simulink model "ClosedLoop_V1_2020b"  (R2020b)
settings: Solver=ode4  StartTime=0.0  StopTime=TMax  FixedStep=DT  MaxStep=DT  RelTol=1e-3  EnableMultiTasking=on
undefined symbols (not defined in the file or in its folder): CertificationSettings, Control, DiscIntNeverNeededParam, Drivetrain, OutList, P_InitAngle, RPM_Init, sigbuilder_block, SimConfig, strmatch
libraries: simulink x10, simulink_extras x4
(part 2 of 2)

== system ClosedLoop_V1_2020b/Plot aerodynamic Data/Plot Reynolds number ==
  note: B1N1Re      Reynolds number (in millions) at Blade 1, Node 1
      | B1N2Re      Reynolds number (in millions) at Blade 1, Node 2
      | B1N3Re      Reynolds number (in millions) at Blade 1, Node 3
      | B1N4Re      Reynolds number (in millions) at Blade 1, Node 4
      | B1N5Re      Reynolds number (in millions) at Blade 1, Node 5
      | B1N6Re      Reynolds number (in millions) at Blade 1, Node 6
      | B1N7Re      Reynolds number (in millions) at Blade 1, Node 7
      | B1N8Re      Reynolds number (in millions) at Blade 1, Node 8
      | B1N9Re      Reynolds number (in millions) at Blade 1, Node 9
  OutData1 : Inport
  Scope : Scope  NumInputPorts=9
  "extract Reynolds number (in millions) at Blade 1, Node 1" : Fcn  Expr=u(strmatch('B1N1Re',OutList))
  "extract Reynolds number (in millions) at Blade 1, Node 2" : Fcn  Expr=u(strmatch('B1N2Re',OutList))
  "extract Reynolds number (in millions) at Blade 1, Node 3" : Fcn  Expr=u(strmatch('B1N3Re',OutList))
  "extract Reynolds number (in millions) at Blade 1, Node 4" : Fcn  Expr=u(strmatch('B1N4Re',OutList))
  "extract Reynolds number (in millions) at Blade 1, Node 5" : Fcn  Expr=u(strmatch('B1N5Re',OutList))
  "extract Reynolds number (in millions) at Blade 1, Node 6" : Fcn  Expr=u(strmatch('B1N6Re',OutList))
  "extract Reynolds number (in millions) at Blade 1, Node 7" : Fcn  Expr=u(strmatch('B1N7Re',OutList))
  "extract Reynolds number (in millions) at Blade 1, Node 8" : Fcn  Expr=u(strmatch('B1N8Re',OutList))
  "extract Reynolds number (in millions) at Blade 1, Node 9" : Fcn  Expr=u(strmatch('B1N9Re',OutList))
  wires:
  OutData1/1 -> "extract Reynolds number (in millions) at Blade 1, Node 9"/1, "extract Reynolds number (in millions) at Blade 1, Node 8"/1, "extract Reynolds number (in millions) at Blade 1, Node 7"/1, "extract Reynolds number (in millions) at Blade 1, Node 6"/1, "extract Reynolds number (in millions) at Blade 1, Node 5"/1, "extract Reynolds number (in millions) at Blade 1, Node 4"/1, "extract Reynolds number (in millions) at Blade 1, Node 3"/1, "extract Reynolds number (in millions) at Blade 1, Node 2"/1, "extract Reynolds number (in millions) at Blade 1, Node 1"/1
  "extract Reynolds number (in millions) at Blade 1, Node 8"/1 -> Scope/8  "Reynolds number (in millions) at Blade 1, Node 8"
  "extract Reynolds number (in millions) at Blade 1, Node 3"/1 -> Scope/3  "Reynolds number (in millions) at Blade 1, Node 3"
  "extract Reynolds number (in millions) at Blade 1, Node 5"/1 -> Scope/5  "Reynolds number (in millions) at Blade 1, Node 5"
  "extract Reynolds number (in millions) at Blade 1, Node 7"/1 -> Scope/7  "Reynolds number (in millions) at Blade 1, Node 7"
  "extract Reynolds number (in millions) at Blade 1, Node 1"/1 -> Scope/1  "Reynolds number (in millions) at Blade 1, Node 1"
  "extract Reynolds number (in millions) at Blade 1, Node 6"/1 -> Scope/6  "Reynolds number (in millions) at Blade 1, Node 6"
  "extract Reynolds number (in millions) at Blade 1, Node 4"/1 -> Scope/4  "Reynolds number (in millions) at Blade 1, Node 4"
  "extract Reynolds number (in millions) at Blade 1, Node 9"/1 -> Scope/9  "Reynolds number (in millions) at Blade 1, Node 9"
  "extract Reynolds number (in millions) at Blade 1, Node 2"/1 -> Scope/2  "Reynolds number (in millions) at Blade 1, Node 2"

== system ClosedLoop_V1_2020b/Plot aerodynamic Data/Plot Rotor Data ==
  note: RtAeroFxh   Total rotor aerodynamic load (force in x direction) the hub coordinate system N
      | RtAeroFyh   Total rotor aerodynamic load (force in y direction) the hub coordinate system N
      | RtAeroFzh   Total rotor aerodynamic load (force in z direction) the hub coordinate system N
      | RtAeroMxh   Total rotor aerodynamic load (moment in x direction) the hub coordinate system Nm
      | RtAeroMyh   Total rotor aerodynamic load (moment in y direction) the hub coordinate system Nm
      | RtAeroMzh   Total rotor aerodynamic load (moment in z direction) the hub coordinate system Nm
      | RtAeroPwr   Rotor aerodynamic power W
      | RtAeroCp    Rotor aerodynamic power coefficient
      | RtAeroCq    Rotor aerodynamic torque coefficient
      | RtAeroCt    Rotor aerodynamic thrust coefficient
  OutData : Inport
  Scope : Scope  NumInputPorts=3
  Scope1 : Scope  NumInputPorts=3
  Scope{2..5} (4 alike) : Scope
  extract Rotor aerodynamic power W : Fcn  Expr=u(strmatch('RtAeroPwr',OutList))
  extract Rotor aerodynamic power coefficient : Fcn  Expr=u(strmatch('RtAeroCp',OutList))
  extract Rotor aerodynamic thrust coefficient : Fcn  Expr=u(strmatch('RtAeroCt',OutList))
  extract Rotor aerodynamic torque coefficient : Fcn  Expr=u(strmatch('RtAeroCp',OutList))
  extract Total rotor aerodynamic load (force in x direction) hub coordinate system (N) : Fcn  Expr=u(strmatch('RtAeroFxh',OutList))
  extract Total rotor aerodynamic load (force in y direction) hub coordinate system (N) : Fcn  Expr=u(strmatch('RtAeroFyh',OutList))
  extract Total rotor aerodynamic load (force in z direction) hub coordinate system (N) : Fcn  Expr=u(strmatch('RtAeroFzh',OutList))
  extract Total rotor aerodynamic load (moment in x direction) the hub coordinate system Nm : Fcn  Expr=u(strmatch('RtAeroMxh',OutList))
  extract Total rotor aerodynamic load (moment in y direction) the hub coordinate system Nm : Fcn  Expr=u(strmatch('RtAeroMyh',OutList))
  extract Total rotor aerodynamic load (moment in z direction) the hub coordinate system Nm : Fcn  Expr=u(strmatch('RtAeroMzh',OutList))
  wires:
  extract Total rotor aerodynamic load (force in x direction) hub coordinate system (N)/1 -> Scope/1  "Total rotor aerodynamic load (force in x direction) hub coordinate system (N)"
  OutData/1 -> extract Rotor aerodynamic thrust coefficient/1, extract Rotor aerodynamic torque coefficient/1, extract Rotor aerodynamic power coefficient/1, extract Rotor aerodynamic power W/1, extract Total rotor aerodynamic load (moment in z direction) the hub coordinate system Nm/1, extract Total rotor aerodynamic load (moment in y direction) the hub coordinate system Nm/1, extract Total rotor aerodynamic load (force in z direction) hub coordinate system (N)/1, extract Total rotor aerodynamic load (force in y direction) hub coordinate system (N)/1, extract Total rotor aerodynamic load (force in x direction) hub coordinate system (N)/1, extract Total rotor aerodynamic load (moment in x direction) the hub coordinate system Nm/1
  extract Total rotor aerodynamic load (force in y direction) hub coordinate system (N)/1 -> Scope/2  "Total rotor aerodynamic load (force in y direction) hub coordinate system (N)"
  extract Total rotor aerodynamic load (force in z direction) hub coordinate system (N)/1 -> Scope/3  "Total rotor aerodynamic load (force in z direction) hub coordinate system (N)"
  extract Total rotor aerodynamic load (moment in x direction) the hub coordinate system Nm/1 -> Scope1/1  "Total rotor aerodynamic load (moment in x direction) the hub coordinate system Nm"
  extract Total rotor aerodynamic load (moment in y direction) the hub coordinate system Nm/1 -> Scope1/2  "Total rotor aerodynamic load (moment in y direction) the hub coordinate system Nm"
  extract Total rotor aerodynamic load (moment in z direction) the hub coordinate system Nm/1 -> Scope1/3  "Total rotor aerodynamic load (moment in z direction) the hub coordinate system Nm"
  extract Rotor aerodynamic power W/1 -> Scope2/1  "Rotor aerodynamic power W"
  extract Rotor aerodynamic power coefficient/1 -> Scope3/1  "Rotor aerodynamic power coefficient"
  extract Rotor aerodynamic torque coefficient/1 -> Scope4/1  "Rotor aerodynamic torque coefficient"
  extract Rotor aerodynamic thrust coefficient/1 -> Scope5/1  "Rotor aerodynamic thrust coefficient"

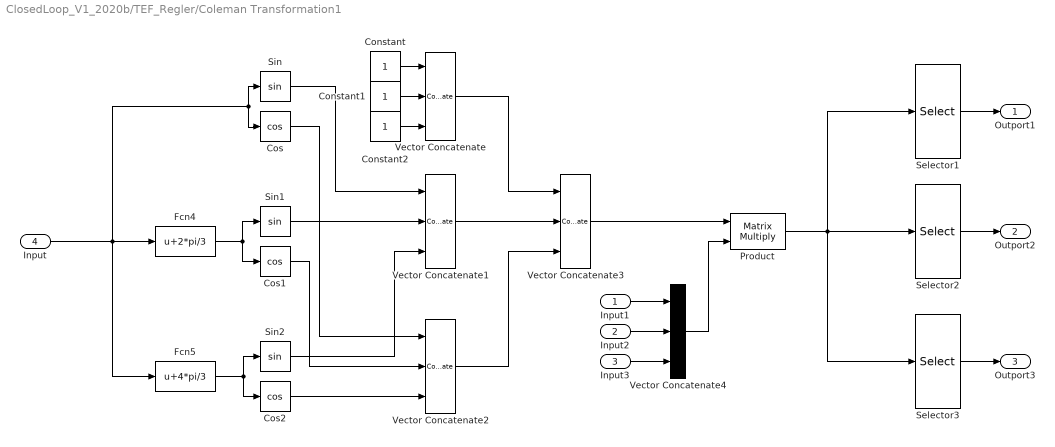
== system ClosedLoop_V1_2020b/TEF_Regler/Coleman Transformation1 ==
  Input1 : Inport
  Input2 : Inport  Port=2
  Input3 : Inport  Port=3
  Input : Inport  Port=4
  Constant : Constant
  Constant1 : Constant
  Constant2 : Constant
  Cos : Trigonometry  Operator=cos
  Cos1 : Trigonometry  Operator=cos
  Cos2 : Trigonometry  Operator=cos
  Fcn4 : Fcn  Expr=u+2*pi/3
  Fcn5 : Fcn  Expr=u+4*pi/3
  Product : Product  Multiplication=Matrix(*)
  Selector1 : Selector  InputPortWidth=3  IndexOptions=Index vector (dialog)  Indices=[1]  OutputSizes=1
  Selector2 : Selector  InputPortWidth=3  IndexOptions=Index vector (dialog)  Indices=[2]  OutputSizes=1
  Selector3 : Selector  InputPortWidth=3  IndexOptions=Index vector (dialog)  Indices=[3]  OutputSizes=1
  Sin : Trigonometry
  Sin1 : Trigonometry
  Sin2 : Trigonometry
  Vector Concatenate{,1..2,4} (4 alike) : Concatenate  NumInputs=3
  Vector Concatenate3 : Concatenate  NumInputs=3  Mode=Multidimensional array  ConcatenateDimension=2
  Outport1 : Outport  VectorParamsAs1DForOutWhenUnconnected=off
  Outport2 : Outport  Port=2  VectorParamsAs1DForOutWhenUnconnected=off
  Outport3 : Outport  Port=3  VectorParamsAs1DForOutWhenUnconnected=off
  wires:
  Input3/1 -> Vector Concatenate4/3
  Input2/1 -> Vector Concatenate4/2
  Input1/1 -> Vector Concatenate4/1
  Constant2/1 -> Vector Concatenate/3
  Vector Concatenate3/1 -> Product/1
  Fcn4/1 -> Cos1/1, Sin1/1
  Vector Concatenate2/1 -> Vector Concatenate3/3
  Selector3/1 -> Outport3/1
  Selector2/1 -> Outport2/1
  Selector1/1 -> Outport1/1
  Vector Concatenate4/1 -> Product/2
  Vector Concatenate1/1 -> Vector Concatenate3/2
  Input/1 -> Cos/1, Sin/1, Fcn4/1, Fcn5/1
  Constant/1 -> Vector Concatenate/1
  Constant1/1 -> Vector Concatenate/2
  Sin2/1 -> Vector Concatenate1/3
  Cos1/1 -> Vector Concatenate2/2
  Cos/1 -> Vector Concatenate2/1
  Sin1/1 -> Vector Concatenate1/2
  Cos2/1 -> Vector Concatenate2/3
  Sin/1 -> Vector Concatenate1/1
  Product/1 -> Selector1/1, Selector2/1, Selector3/1
  Vector Concatenate/1 -> Vector Concatenate3/1
  Fcn5/1 -> Cos2/1, Sin2/1

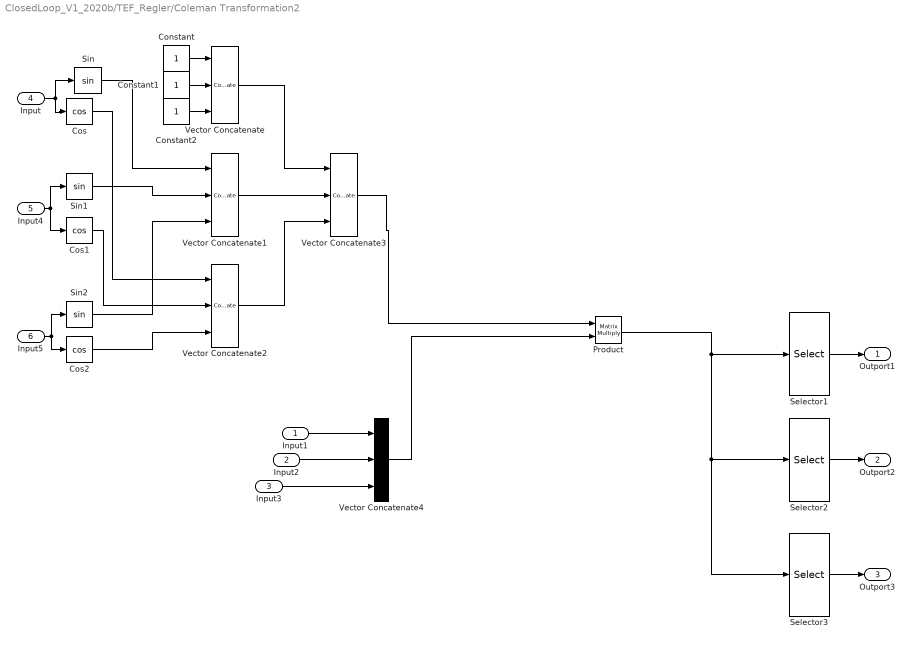
== system ClosedLoop_V1_2020b/TEF_Regler/Coleman Transformation2 ==
  Input1 : Inport
  Input2 : Inport  Port=2
  Input3 : Inport  Port=3
  Input : Inport  Port=4
  Input4 : Inport  Port=5
  Input5 : Inport  Port=6
  Constant : Constant
  Constant1 : Constant
  Constant2 : Constant
  Cos : Trigonometry  Operator=cos
  Cos1 : Trigonometry  Operator=cos
  Cos2 : Trigonometry  Operator=cos
  Product : Product  Multiplication=Matrix(*)
  Selector1 : Selector  InputPortWidth=3  IndexOptions=Index vector (dialog)  Indices=[1]  OutputSizes=1
  Selector2 : Selector  InputPortWidth=3  IndexOptions=Index vector (dialog)  Indices=[2]  OutputSizes=1
  Selector3 : Selector  InputPortWidth=3  IndexOptions=Index vector (dialog)  Indices=[3]  OutputSizes=1
  Sin : Trigonometry
  Sin1 : Trigonometry
  Sin2 : Trigonometry
  Vector Concatenate{,1..2,4} (4 alike) : Concatenate  NumInputs=3
  Vector Concatenate3 : Concatenate  NumInputs=3  Mode=Multidimensional array  ConcatenateDimension=2
  Outport1 : Outport  VectorParamsAs1DForOutWhenUnconnected=off
  Outport2 : Outport  Port=2  VectorParamsAs1DForOutWhenUnconnected=off
  Outport3 : Outport  Port=3  VectorParamsAs1DForOutWhenUnconnected=off
  wires:
  Input3/1 -> Vector Concatenate4/3
  Input2/1 -> Vector Concatenate4/2
  Input1/1 -> Vector Concatenate4/1
  Constant2/1 -> Vector Concatenate/3
  Vector Concatenate3/1 -> Product/1
  Input4/1 -> Sin1/1, Cos1/1
  Vector Concatenate2/1 -> Vector Concatenate3/3
  Selector3/1 -> Outport3/1
  Selector2/1 -> Outport2/1
  Selector1/1 -> Outport1/1
  Vector Concatenate4/1 -> Product/2
  Vector Concatenate1/1 -> Vector Concatenate3/2
  Input5/1 -> Sin2/1, Cos2/1
  Constant/1 -> Vector Concatenate/1
  Constant1/1 -> Vector Concatenate/2
  Sin2/1 -> Vector Concatenate1/3
  Cos1/1 -> Vector Concatenate2/2
  Cos/1 -> Vector Concatenate2/1
  Sin1/1 -> Vector Concatenate1/2
  Cos2/1 -> Vector Concatenate2/3
  Sin/1 -> Vector Concatenate1/1
  Input/1 -> Sin/1, Cos/1
  Product/1 -> Selector1/1, Selector2/1, Selector3/1
  Vector Concatenate/1 -> Vector Concatenate3/1

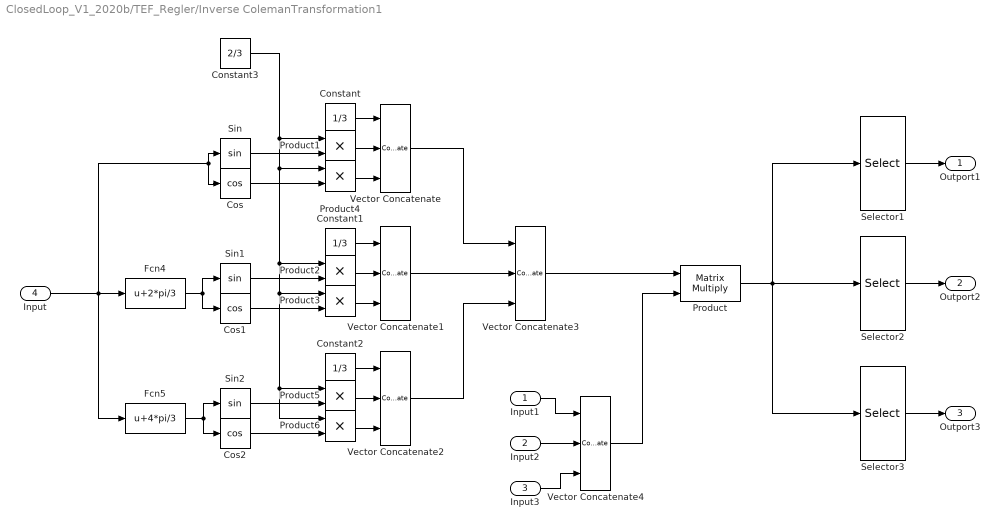
== system ClosedLoop_V1_2020b/TEF_Regler/Inverse ColemanTransformation1 ==
  Input1 : Inport
  Input2 : Inport  Port=2
  Input3 : Inport  Port=3
  Input : Inport  Port=4
  Constant : Constant  Value=1/3
  Constant1 : Constant  Value=1/3
  Constant2 : Constant  Value=1/3
  Constant3 : Constant  Value=2/3
  Cos : Trigonometry  Operator=cos
  Cos1 : Trigonometry  Operator=cos
  Cos2 : Trigonometry  Operator=cos
  Fcn4 : Fcn  Expr=u+2*pi/3
  Fcn5 : Fcn  Expr=u+4*pi/3
  Product : Product  Multiplication=Matrix(*)
  Product{1..6} (6 alike) : Product
  Selector1 : Selector  InputPortWidth=3  IndexOptions=Index vector (dialog)  Indices=[1]  OutputSizes=1
  Selector2 : Selector  InputPortWidth=3  IndexOptions=Index vector (dialog)  Indices=[2]  OutputSizes=1
  Selector3 : Selector  InputPortWidth=3  IndexOptions=Index vector (dialog)  Indices=[3]  OutputSizes=1
  Sin : Trigonometry
  Sin1 : Trigonometry
  Sin2 : Trigonometry
  Vector Concatenate{,1..2,4} (4 alike) : Concatenate  NumInputs=3  Mode=Multidimensional array
  Vector Concatenate3 : Concatenate  NumInputs=3  Mode=Multidimensional array  ConcatenateDimension=2
  Outport1 : Outport  VectorParamsAs1DForOutWhenUnconnected=off
  Outport2 : Outport  Port=2  VectorParamsAs1DForOutWhenUnconnected=off
  Outport3 : Outport  Port=3  VectorParamsAs1DForOutWhenUnconnected=off
  wires:
  Selector2/1 -> Outport2/1
  Selector3/1 -> Outport3/1
  Product/1 -> Selector1/1, Selector2/1, Selector3/1
  Selector1/1 -> Outport1/1
  Product2/1 -> Vector Concatenate1/2
  Product1/1 -> Vector Concatenate/2
  Constant/1 -> Vector Concatenate/1
  Vector Concatenate1/1 -> Vector Concatenate3/2
  Vector Concatenate2/1 -> Vector Concatenate3/3
  Vector Concatenate/1 -> Vector Concatenate3/1
  Vector Concatenate3/1 -> Product/1
  Input/1 -> Fcn4/1, Fcn5/1, Cos/1, Sin/1
  Product4/1 -> Vector Concatenate/3
  Sin1/1 -> Product2/2
  Constant1/1 -> Vector Concatenate1/1
  Product6/1 -> Vector Concatenate2/3
  Constant2/1 -> Vector Concatenate2/1
  Product3/1 -> Vector Concatenate1/3
  Sin/1 -> Product1/2
  Product5/1 -> Vector Concatenate2/2
  Input3/1 -> Vector Concatenate4/3
  Vector Concatenate4/1 -> Product/2
  Input1/1 -> Vector Concatenate4/1
  Input2/1 -> Vector Concatenate4/2
  Constant3/1 -> Product4/1, Product2/1, Product6/1, Product5/1, Product3/1, Product1/1
  Cos/1 -> Product4/2
  Cos1/1 -> Product3/2
  Sin2/1 -> Product5/2
  Cos2/1 -> Product6/2
  Fcn4/1 -> Sin1/1, Cos1/1
  Fcn5/1 -> Sin2/1, Cos2/1

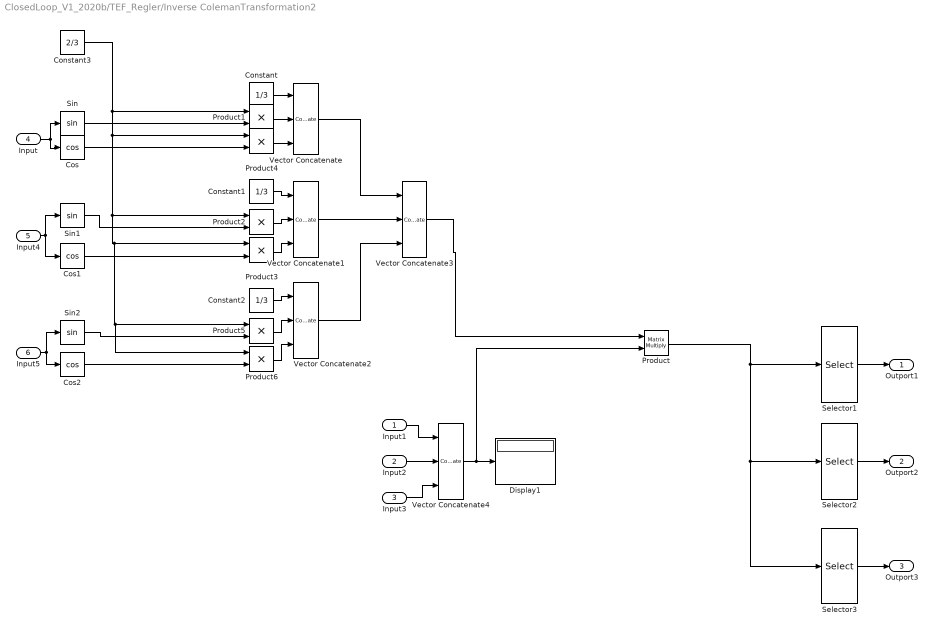
== system ClosedLoop_V1_2020b/TEF_Regler/Inverse ColemanTransformation2 ==
  Input1 : Inport
  Input2 : Inport  Port=2
  Input3 : Inport  Port=3
  Input : Inport  Port=4
  Input4 : Inport  Port=5
  Input5 : Inport  Port=6
  Constant : Constant  Value=1/3
  Constant1 : Constant  Value=1/3
  Constant2 : Constant  Value=1/3
  Constant3 : Constant  Value=2/3
  Cos : Trigonometry  Operator=cos
  Cos1 : Trigonometry  Operator=cos
  Cos2 : Trigonometry  Operator=cos
  Display1 : Display
  Product : Product  Multiplication=Matrix(*)
  Product{1..6} (6 alike) : Product
  Selector1 : Selector  InputPortWidth=3  IndexOptions=Index vector (dialog)  Indices=[1]  OutputSizes=1
  Selector2 : Selector  InputPortWidth=3  IndexOptions=Index vector (dialog)  Indices=[2]  OutputSizes=1
  Selector3 : Selector  InputPortWidth=3  IndexOptions=Index vector (dialog)  Indices=[3]  OutputSizes=1
  Sin : Trigonometry
  Sin1 : Trigonometry
  Sin2 : Trigonometry
  Vector Concatenate{,1..2,4} (4 alike) : Concatenate  NumInputs=3  Mode=Multidimensional array
  Vector Concatenate3 : Concatenate  NumInputs=3  Mode=Multidimensional array  ConcatenateDimension=2
  Outport1 : Outport  VectorParamsAs1DForOutWhenUnconnected=off
  Outport2 : Outport  Port=2  VectorParamsAs1DForOutWhenUnconnected=off
  Outport3 : Outport  Port=3  VectorParamsAs1DForOutWhenUnconnected=off
  wires:
  Selector2/1 -> Outport2/1
  Selector3/1 -> Outport3/1
  Product/1 -> Selector1/1, Selector2/1, Selector3/1
  Selector1/1 -> Outport1/1
  Input4/1 -> Sin1/1, Cos1/1
  Product2/1 -> Vector Concatenate1/2
  Product1/1 -> Vector Concatenate/2
  Constant/1 -> Vector Concatenate/1
  Vector Concatenate1/1 -> Vector Concatenate3/2
  Vector Concatenate2/1 -> Vector Concatenate3/3
  Input/1 -> Cos/1, Sin/1
  Vector Concatenate/1 -> Vector Concatenate3/1
  Vector Concatenate3/1 -> Product/1
  Input5/1 -> Sin2/1, Cos2/1
  Product4/1 -> Vector Concatenate/3
  Sin1/1 -> Product2/2
  Constant1/1 -> Vector Concatenate1/1
  Product6/1 -> Vector Concatenate2/3
  Constant2/1 -> Vector Concatenate2/1
  Product3/1 -> Vector Concatenate1/3
  Sin/1 -> Product1/2
  Product5/1 -> Vector Concatenate2/2
  Input3/1 -> Vector Concatenate4/3
  Vector Concatenate4/1 -> Display1/1, Product/2
  Input1/1 -> Vector Concatenate4/1
  Input2/1 -> Vector Concatenate4/2
  Constant3/1 -> Product1/1, Product4/1, Product2/1, Product3/1, Product5/1, Product6/1
  Cos/1 -> Product4/2
  Cos1/1 -> Product3/2
  Sin2/1 -> Product5/2
  Cos2/1 -> Product6/2

== system ClosedLoop_V1_2020b/TEF_Regler/Subsystem ==
  In1 : Inport
  Derivative : Derivative
  Gain : Gain  Gain=SimConfig.controller.TEF.K_P
  Gain1 : Gain  Gain=SimConfig.controller.TEF.K_I
  Gain2 : Gain  Gain=SimConfig.controller.TEF.K_D
  Integrator : Integrator
  Scope : Scope  NumInputPorts=2
  Scope1 : Scope  NumInputPorts=2
  Scope2 : Scope  NumInputPorts=5
  Sum : Sum  Inputs=+++
  Out1 : Outport  VectorParamsAs1DForOutWhenUnconnected=off
  wires:
  Sum/1 -> Scope2/4, Out1/1
  Integrator/1 -> Gain1/1  "I"
  Derivative/1 -> Gain2/1
  In1/1 -> Scope2/5, Scope/1, Gain/1, Scope1/2, Integrator/1, Derivative/1
  Gain/1 -> Scope/2, Scope2/2, Sum/2  "P"
  Gain1/1 -> Scope1/1, Scope2/3, Sum/3
  Gain2/1 -> Sum/1, Scope2/1  "D"

== system ClosedLoop_V1_2020b/TEF_Regler/Subsystem1 ==
  In1 : Inport
  Derivative : Derivative
  Gain : Gain  Gain=SimConfig.controller.TEF.K_P
  Gain1 : Gain  Gain=SimConfig.controller.TEF.K_I
  Gain2 : Gain  Gain=SimConfig.controller.TEF.K_D
  Integrator : Integrator
  Sum : Sum  Inputs=+++
  Out1 : Outport  VectorParamsAs1DForOutWhenUnconnected=off
  wires:
  Gain2/1 -> Sum/1
  Gain1/1 -> Sum/3
  Gain/1 -> Sum/2
  In1/1 -> Derivative/1, Integrator/1, Gain/1
  Derivative/1 -> Gain2/1
  Integrator/1 -> Gain1/1
  Sum/1 -> Out1/1

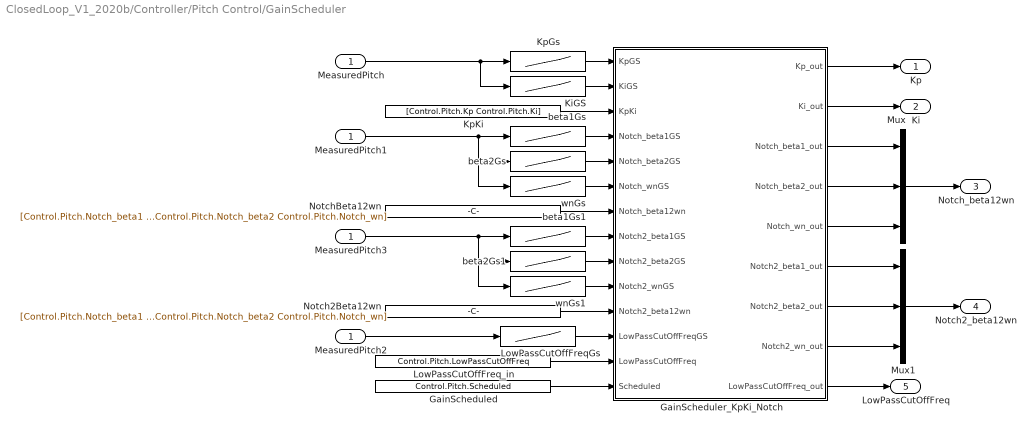
== system ClosedLoop_V1_2020b/Controller/Pitch Control/GainScheduler ==
  MeasuredPitch : Inport
  GainScheduled : Constant  Value=Control.Pitch.Scheduled
  GainScheduler_KpKi_Notch : MATLAB Function  TreatAsAtomicUnit=on
  KiGS : Lookup_n-D  NumberOfTableDimensions=1  BreakpointsForDimension1=Control.Pitch.ScheduledPitchAngles  Table=Control.Pitch.KiGS  ExtrapMethod=Clip  UseLastTableValue=on  InternalRulePriority=Speed  RndMeth=Simplest  InputSameDT=on
  KpGs : Lookup_n-D  NumberOfTableDimensions=1  BreakpointsForDimension1=Control.Pitch.ScheduledPitchAngles  Table=Control.Pitch.KpGS  ExtrapMethod=Clip  UseLastTableValue=on  InternalRulePriority=Speed  RndMeth=Simplest  InputSameDT=on
  KpKi : Constant  Value=[Control.Pitch.Kp Control.Pitch.Ki]
  LowPassCutOffFreqGs : Lookup_n-D  NumberOfTableDimensions=1  BreakpointsForDimension1=Control.Pitch.ScheduledPitchAngles  Table=Control.Pitch.LowPassCutOffFreqGS  ExtrapMethod=Clip  UseLastTableValue=on  InternalRulePriority=Speed  RndMeth=Simplest  InputSameDT=on
  LowPassCutOffFreq_in : Constant  Value=Control.Pitch.LowPassCutOffFreq
  MeasuredPitch1 : InportShadow
  MeasuredPitch2 : InportShadow
  MeasuredPitch3 : InportShadow
  Mux : Mux  Inputs=3
  Mux1 : Mux  Inputs=3
  Notch2Beta12wn : Constant  Value=[Control.Pitch.Notch_beta1 Control.Pitch.Notch_beta2 Control.Pitch.Notch_wn]
  NotchBeta12wn : Constant  Value=[Control.Pitch.Notch_beta1 Control.Pitch.Notch_beta2 Control.Pitch.Notch_wn]
  beta1Gs : Lookup_n-D  NumberOfTableDimensions=1  BreakpointsForDimension1=Control.Pitch.ScheduledPitchAngles  Table=Control.Pitch.Notch_beta1GS  ExtrapMethod=Clip  UseLastTableValue=on  InternalRulePriority=Speed  RndMeth=Simplest  InputSameDT=on
  beta1Gs1 : Lookup_n-D  NumberOfTableDimensions=1  BreakpointsForDimension1=Control.Pitch.ScheduledPitchAngles  Table=Control.Pitch.Notch2_beta1GS  ExtrapMethod=Clip  UseLastTableValue=on  InternalRulePriority=Speed  RndMeth=Simplest  InputSameDT=on
  beta2Gs : Lookup_n-D  NumberOfTableDimensions=1  BreakpointsForDimension1=Control.Pitch.ScheduledPitchAngles  Table=Control.Pitch.Notch_beta2GS  ExtrapMethod=Clip  UseLastTableValue=on  InternalRulePriority=Speed  RndMeth=Simplest  InputSameDT=on
  beta2Gs1 : Lookup_n-D  NumberOfTableDimensions=1  BreakpointsForDimension1=Control.Pitch.ScheduledPitchAngles  Table=Control.Pitch.Notch2_beta2GS  ExtrapMethod=Clip  UseLastTableValue=on  InternalRulePriority=Speed  RndMeth=Simplest  InputSameDT=on
  wnGs : Lookup_n-D  NumberOfTableDimensions=1  BreakpointsForDimension1=Control.Pitch.ScheduledPitchAngles  Table=Control.Pitch.Notch_wnGS  ExtrapMethod=Clip  UseLastTableValue=on  InternalRulePriority=Speed  RndMeth=Simplest  InputSameDT=on
  wnGs1 : Lookup_n-D  NumberOfTableDimensions=1  BreakpointsForDimension1=Control.Pitch.ScheduledPitchAngles  Table=Control.Pitch.Notch2_wnGS  ExtrapMethod=Clip  UseLastTableValue=on  InternalRulePriority=Speed  RndMeth=Simplest  InputSameDT=on
  Kp : Outport  VectorParamsAs1DForOutWhenUnconnected=off
  Ki : Outport  Port=2  VectorParamsAs1DForOutWhenUnconnected=off
  Notch_beta12wn : Outport  Port=3  VectorParamsAs1DForOutWhenUnconnected=off
  Notch2_beta12wn : Outport  Port=4  VectorParamsAs1DForOutWhenUnconnected=off
  LowPassCutOffFreq : Outport  Port=5  VectorParamsAs1DForOutWhenUnconnected=off
  wires:
  MeasuredPitch/1 -> KiGS/1, KpGs/1
  GainScheduled/1 -> GainScheduler_KpKi_Notch/14(Scheduled)
  GainScheduler_KpKi_Notch/2(Ki_out) -> Ki/1
  KpKi/1 -> GainScheduler_KpKi_Notch/3(KpKi)
  KpGs/1 -> GainScheduler_KpKi_Notch/1(KpGS)
  KiGS/1 -> GainScheduler_KpKi_Notch/2(KiGS)
  GainScheduler_KpKi_Notch/1(Kp_out) -> Kp/1
  GainScheduler_KpKi_Notch/3(Notch_beta1_out) -> Mux/1
  GainScheduler_KpKi_Notch/4(Notch_beta2_out) -> Mux/2
  GainScheduler_KpKi_Notch/5(Notch_wn_out) -> Mux/3
  NotchBeta12wn/1 -> GainScheduler_KpKi_Notch/7(Notch_beta12wn)
  MeasuredPitch1/1 -> wnGs/1, beta2Gs/1, beta1Gs/1
  beta1Gs/1 -> GainScheduler_KpKi_Notch/4(Notch_beta1GS)
  beta2Gs/1 -> GainScheduler_KpKi_Notch/5(Notch_beta2GS)
  wnGs/1 -> GainScheduler_KpKi_Notch/6(Notch_wnGS)
  Mux/1 -> Notch_beta12wn/1
  MeasuredPitch2/1 -> LowPassCutOffFreqGs/1
  LowPassCutOffFreqGs/1 -> GainScheduler_KpKi_Notch/12(LowPassCutOffFreqGS)
  LowPassCutOffFreq_in/1 -> GainScheduler_KpKi_Notch/13(LowPassCutOffFreq)
  GainScheduler_KpKi_Notch/9(LowPassCutOffFreq_out) -> LowPassCutOffFreq/1
  GainScheduler_KpKi_Notch/7(Notch2_beta2_out) -> Mux1/2
  Mux1/1 -> Notch2_beta12wn/1
  GainScheduler_KpKi_Notch/6(Notch2_beta1_out) -> Mux1/1
  GainScheduler_KpKi_Notch/8(Notch2_wn_out) -> Mux1/3
  MeasuredPitch3/1 -> wnGs1/1, beta2Gs1/1, beta1Gs1/1
  beta1Gs1/1 -> GainScheduler_KpKi_Notch/8(Notch2_beta1GS)
  beta2Gs1/1 -> GainScheduler_KpKi_Notch/9(Notch2_beta2GS)
  wnGs1/1 -> GainScheduler_KpKi_Notch/10(Notch2_wnGS)
  Notch2Beta12wn/1 -> GainScheduler_KpKi_Notch/11(Notch2_beta12wn)

== system ClosedLoop_V1_2020b/Controller/Pitch Control/Low-pass filter ==
  LowPassCutOffFreq : Inport
  u : Inport  Port=2
  Constant : Constant  Value=Control.DT
  Constant1 : Constant  Value=1/sqrt(2)
  Constant2 : Constant  Value=Control.Pitch.LowPassOrder
  Constant3 : Constant  Value=Control.DT
  First-order low-pass filter : MATLAB Function  TreatAsAtomicUnit=on
  Second-order low-pass filter : MATLAB Function  TreatAsAtomicUnit=on
  Switch : Switch  Criteria=u2 > Threshold  Threshold=1.5
  Output : Outport  VectorParamsAs1DForOutWhenUnconnected=off
  wires:
  Switch/1 -> Output/1
  Constant1/1 -> Second-order low-pass filter/3(Damp)
  Constant/1 -> Second-order low-pass filter/4(Ts)
  Constant3/1 -> First-order low-pass filter/3(Ts)
  Constant2/1 -> Switch/2
  First-order low-pass filter/1(y) -> Switch/3
  Second-order low-pass filter/1(y) -> Switch/1
  LowPassCutOffFreq/1 -> Second-order low-pass filter/2(wn), First-order low-pass filter/2(wn)
  u/1 -> First-order low-pass filter/1(u), Second-order low-pass filter/1(u)

== system ClosedLoop_V1_2020b/Controller/Pitch Control/Notch filter ==
  u : Inport
  beta12wn : Inport  Port=2
  Constant : Constant  Value=Control.DT
  Demux : Demux  Outputs=3
  MATLAB Function : MATLAB Function  TreatAsAtomicUnit=on
  Out1 : Outport  VectorParamsAs1DForOutWhenUnconnected=off
  wires:
  MATLAB Function/1(y) -> Out1/1
  Demux/1 -> MATLAB Function/2(beta1)
  Demux/2 -> MATLAB Function/3(beta2)
  Demux/3 -> MATLAB Function/4(wn)
  beta12wn/1 -> Demux/1
  u/1 -> MATLAB Function/1(u)
  Constant/1 -> MATLAB Function/5(Ts)

== system ClosedLoop_V1_2020b/Controller/Pitch Control/Notch filter1 ==
  u : Inport
  beta12wn : Inport  Port=2
  Constant : Constant  Value=Control.DT
  Demux : Demux  Outputs=3
  MATLAB Function : MATLAB Function  TreatAsAtomicUnit=on
  Out1 : Outport  VectorParamsAs1DForOutWhenUnconnected=off
  wires:
  MATLAB Function/1(y) -> Out1/1
  Demux/1 -> MATLAB Function/2(beta1)
  Demux/2 -> MATLAB Function/3(beta2)
  Demux/3 -> MATLAB Function/4(wn)
  beta12wn/1 -> Demux/1
  u/1 -> MATLAB Function/1(u)
  Constant/1 -> MATLAB Function/5(Ts)

== system ClosedLoop_V1_2020b/Controller/Torque Control/Low-pass filter ==
  u : Inport
  Constant1 : Constant  Value=Control.Torque.LowPassCutOffFreq
  Constant3 : Constant  Value=Control.DT
  First-order low-pass filter : MATLAB Function  TreatAsAtomicUnit=on
  Output : Outport  VectorParamsAs1DForOutWhenUnconnected=off
  wires:
  Constant3/1 -> First-order low-pass filter/3(Ts)
  u/1 -> First-order low-pass filter/1(u)
  First-order low-pass filter/1(y) -> Output/1
  Constant1/1 -> First-order low-pass filter/2(wn)

== matlab function ClosedLoop_V1_2020b/Controller/Pitch Control/GainScheduler/GainScheduler_KpKi_Notch ==
  data: KpGS input; KiGS input; Kp_out output; KpKi input; Notch_beta1GS input; Notch_beta2GS input; Notch_wnGS input; Notch_beta12wn input; Notch2_beta1GS input; Notch2_beta2GS input; Notch2_wnGS input; Notch2_beta12wn input; LowPassCutOffFreqGS input; LowPassCutOffFreq input; Scheduled input; Ki_out output; Notch_beta1_out output; Notch_beta2_out output; Notch_wn_out output; Notch2_beta1_out output; Notch2_beta2_out output; Notch2_wn_out output; LowPassCutOffFreq_out output
function [Kp_out, Ki_out, Notch_beta1_out, Notch_beta2_out, Notch_wn_out, Notch2_beta1_out, Notch2_beta2_out, Notch2_wn_out, LowPassCutOffFreq_out] = fcn(KpGS, KiGS, KpKi, Notch_beta1GS, Notch_beta2GS, Notch_wnGS, Notch_beta12wn, Notch2_beta1GS, Notch2_beta2GS, Notch2_wnGS, Notch2_beta12wn, LowPassCutOffFreqGS, LowPassCutOffFreq, Scheduled)

if Scheduled > 0.5
    Kp_out = KpGS;
    Ki_out = KiGS;
    Notch_beta1_out = Notch_beta1GS;
    Notch_beta2_out = Notch_beta2GS;
    Notch_wn_out = Notch_wnGS;
    Notch2_beta1_out = Notch2_beta1GS;
    Notch2_beta2_out = Notch2_beta2GS;
    Notch2_wn_out = Notch2_wnGS;
    LowPassCutOffFreq_out = LowPassCutOffFreqGS;
else
    Kp_out = KpKi(1);
    Ki_out = KpKi(2);
    Notch_beta1_out = Notch_beta12wn(1);
    Notch_beta2_out = Notch_beta12wn(2);
    Notch_wn_out = Notch_beta12wn(3);
    Notch2_beta1_out = Notch2_beta12wn(1);
    Notch2_beta2_out = Notch2_beta12wn(2);
    Notch2_wn_out = Notch2_beta12wn(3);
    LowPassCutOffFreq_out = LowPassCutOffFreq;
end

== matlab function ClosedLoop_V1_2020b/Controller/Pitch Control/Notch filter/MATLAB Function ==
  data: u input; beta1 input; beta2 input; wn input; y output; Ts input
function y = NotchFilter(u, beta1, beta2, wn, Ts)

persistent u_prev1 u_prev2 y_prev1 y_prev2
if isempty(u_prev1)
    u_prev1 = u;
    u_prev2 = u;
    y_prev1 = u;
    y_prev2 = u;
end

if any([beta1 beta2 wn] == 0)
    y = u;
else
    % Prepare filter elements from current input
    K = 2/Ts;
    Part1 = (K^2 + 2*wn*beta1 * K + wn^2) / (K^2 + 2*wn*beta2 * K + wn^2);
    Part2 = (2 * wn^2 - 2 * K^2)  / (K^2 + 2*wn*beta2 * K + wn^2);
    Part3 = (K^2 - 2*wn*beta1 * K + wn^2) / (K^2 + 2*wn*beta2 * K + wn^2);
    Part4 = (2 * wn^2 - 2 * K^2)  / (K^2 + 2*wn*beta2 * K + wn^2);
    Part5 = (K^2 - 2*wn*beta2* K + wn^2)/ (K^2 + 2*wn*beta2 * K + wn^2);
    
    % Compute filter output
    y = Part1*u + Part2*u_prev1 + Part3*u_prev2 - Part4*y_prev1 - Part5*y_prev2;
    
    % Save signals for next time step
    u_prev2 = u_prev1;
    u_prev1 = u;
    
    y_prev2 = y_prev1;
    y_prev1 = y;
end

== matlab function ClosedLoop_V1_2020b/Controller/Pitch Control/Low-pass filter/Second-order low-pass filter ==
  data: u input; wn input; Damp input; y output; Ts input
function y = SecLPF(u, wn, Damp, Ts)

persistent y_prev1 y_prev2 u_prev1 u_prev2

if isempty(u_prev1)
    y_prev1 = u;
    y_prev2 = u;
    u_prev1 = u;
    u_prev2 = u;
end

y = 1/(4+4*Ts*Damp*wn+Ts^2*wn^2) * ( (8-2*Ts^2*wn^2)*y_prev1 + ...
    (-4+4*Ts*Damp*wn-Ts^2*wn^2)*y_prev2 + (Ts^2*wn^2)*u ...
    + (2*Ts^2*wn^2)*u_prev1 + (Ts^2*wn^2)*u_prev2 );

u_prev2   = u_prev1;
u_prev1   = u;
y_prev2  = y_prev1;
y_prev1  = y;

== matlab function ClosedLoop_V1_2020b/Controller/Pitch Control/Low-pass filter/First-order low-pass filter ==
  data: u input; wn input; y output; Ts input
function y = FirstLPF(u, wn, Ts)

persistent y_prev1 u_prev1

if isempty(u_prev1)
    y_prev1 = u;
    u_prev1 = u;
end

y = (Ts*wn*u + Ts*wn*u_prev1 - (Ts*wn-2.0)*y_prev1)/(Ts*wn+2.0);

u_prev1   = u;
y_prev1  = y;

== matlab function ClosedLoop_V1_2020b/Controller/Rate Saturation Torque ==
  settings: updateMethod=DISCRETE
  data: u input; MinSaturation input; y_out output; MaxSaturation input; DT input
function y_out = fcn(u, MinSaturation, MaxSaturation, DT)
persistent y

if isempty(y)
    y = u;
end

rate = (u-y)/DT;
rate = min(max(rate, MinSaturation), MaxSaturation);

y = y + rate*DT;
y_out = y;

== matlab function ClosedLoop_V1_2020b/Controller/Pitch Control/Notch filter1/MATLAB Function ==
  data: u input; beta1 input; beta2 input; wn input; y output; Ts input
function y = NotchFilter(u, beta1, beta2, wn, Ts)

persistent u_prev1 u_prev2 y_prev1 y_prev2
if isempty(u_prev1)
    u_prev1 = u;
    u_prev2 = u;
    y_prev1 = u;
    y_prev2 = u;
end

if any([beta1 beta2 wn] == 0)
    y = u;
else
    % Prepare filter elements from current input
    K = 2/Ts;
    Part1 = (K^2 + 2*wn*beta1 * K + wn^2) / (K^2 + 2*wn*beta2 * K + wn^2);
    Part2 = (2 * wn^2 - 2 * K^2)  / (K^2 + 2*wn*beta2 * K + wn^2);
    Part3 = (K^2 - 2*wn*beta1 * K + wn^2) / (K^2 + 2*wn*beta2 * K + wn^2);
    Part4 = (2 * wn^2 - 2 * K^2)  / (K^2 + 2*wn*beta2 * K + wn^2);
    Part5 = (K^2 - 2*wn*beta2* K + wn^2)/ (K^2 + 2*wn*beta2 * K + wn^2);
    
    % Compute filter output
    y = Part1*u + Part2*u_prev1 + Part3*u_prev2 - Part4*y_prev1 - Part5*y_prev2;
    
    % Save signals for next time step
    u_prev2 = u_prev1;
    u_prev1 = u;
    
    y_prev2 = y_prev1;
    y_prev1 = y;
end

== matlab function ClosedLoop_V1_2020b/Controller/Torque Control/Low-pass filter/First-order low-pass filter ==
  data: u input; wn input; y output; Ts input
function y = FirstLPF(u, wn, Ts)

persistent y_prev1 u_prev1

if isempty(u_prev1)
    y_prev1 = u;
    u_prev1 = u;
end

y = (Ts*wn*u + Ts*wn*u_prev1 - (Ts*wn-2.0)*y_prev1)/(Ts*wn+2.0);

u_prev1   = u;
y_prev1  = y;

== matlab function ClosedLoop_V1_2020b/Controller/Torque Control/TorqueController ==
  data: GeneratorTorqueDemand output; MeasuredGeneratorSpeed input; MeasuredPitch input; Control_Torque_OptGain input; omega_ABCD input size=[1 4]; P_StartupMode input; Torque_Demanded input; FineMaxPitch input; T_MinTorque input; Clock input; Event input; EventTime input
function GeneratorTorqueDemand  = TorqueController(MeasuredGeneratorSpeed, MeasuredPitch, Control_Torque_OptGain, omega_ABCD, P_StartupMode, Torque_Demanded, FineMaxPitch, T_MinTorque, Clock, Event, EventTime)

% Calculate generator torque setpoint according to the feedforward wind
% turbine control law T = K*\omega^2
GeneratorTorqueDemand = max(min(Control_Torque_OptGain*MeasuredGeneratorSpeed^2, Torque_Demanded), T_MinTorque);

% Calculate torques at beginning and end of CP_max operation
TorqueOmegaB = Control_Torque_OptGain*(omega_ABCD(2)*pi/30)^2;
TorqueOmegaC = Control_Torque_OptGain*(omega_ABCD(3)*pi/30)^2;

% Apply maximum demanded torque when pitch is 1 degree above fine-pitch and
% the wind turbine is not in start-up mode.
if (Event == 5 && Clock >= EventTime) && (MeasuredPitch > (FineMaxPitch(2) - 1.0)*pi/180) %Emergency shutdown
    GeneratorTorqueDemand = 0.0;
elseif MeasuredPitch > (FineMaxPitch(1) + 1.0)*pi/180 && P_StartupMode == false
    GeneratorTorqueDemand = Torque_Demanded;
elseif MeasuredGeneratorSpeed < omega_ABCD(1)*pi/30
    GeneratorTorqueDemand = T_MinTorque;
elseif MeasuredGeneratorSpeed < omega_ABCD(2)*pi/30
    GeneratorTorqueDemand = (TorqueOmegaB - T_MinTorque)/((omega_ABCD(2) - omega_ABCD(1))*pi/30)*(MeasuredGeneratorSpeed - omega_ABCD(1)*pi/30) + T_MinTorque;
elseif MeasuredGeneratorSpeed >= omega_ABCD(3)*pi/30
    GeneratorTorqueDemand = (Torque_Demanded - TorqueOmegaC)/((omega_ABCD(4) - omega_ABCD(3))*pi/30)*(MeasuredGeneratorSpeed - omega_ABCD(3)*pi/30) + TorqueOmegaC;
end

== matlab function ClosedLoop_V1_2020b/MATLAB Function2 ==
  data: switch_signal input; Output output; Input_1 input; Input_2 input
function Output  = fcn(switch_signal, Input_1, Input_2)

if switch_signal == 1
    Output = Input_1;
else
    Output = Input_2;
end

== matlab function ClosedLoop_V1_2020b/Individual Pitch Controller/MBC ==
  data: M1 input; M_N2 output; M2 input; M3 input; Phi input; M_N3 output
function [M_N2, M_N3] = fcn(M1,M2,M3,Phi)

M_N2 = 2/3 * cos(Phi) * M1 + 2/3 * cos(Phi+2*pi/3) * M2 + 2/3 * cos(Phi+4*pi/3) * M3;
M_N3 = 2/3 * sin(Phi) * M1 + 2/3 * sin(Phi+2*pi/3) * M2 + 2/3 * sin(Phi+4*pi/3) * M3;

== matlab function ClosedLoop_V1_2020b/Individual Pitch Controller/Inverse MBC ==
  data: M_N2 input; beta output; M_N3 input; Phi input
function beta  = fcn(M_N2,M_N3,Phi)

beta_1 = cos(Phi) * M_N2 + sin(Phi) * M_N3;
beta_2 = cos(Phi+2*pi/3) * M_N2 + sin(Phi+2*pi/3) * M_N3;
beta_3 = cos(Phi+4*pi/3) * M_N2 + sin(Phi+4*pi/3) * M_N3;

beta = [beta_1,beta_2,beta_3];

== matlab function ClosedLoop_V1_2020b/Individual Pitch Controller/Rate Saturation Pitch ==
  settings: updateMethod=DISCRETE
  data: u input; MinSaturation input; y_out output; MaxSaturation input; DT input
function y_out = fcn(u, MinSaturation, MaxSaturation, DT)
persistent y

if isempty(y)
    y = u;
end

rate = (u-y)/DT;
rate = min(max(rate, MinSaturation), MaxSaturation);

y = y + rate*DT;
y_out = y;

== matlab function ClosedLoop_V1_2020b/MATLAB Function3 ==
  data: switch_signal input; Output output; Input_1 input; Input_2 input
function Output  = fcn(switch_signal, Input_1, Input_2)

if switch_signal == 1
    Output = Input_1;
else
    Output = Input_2;
end

== matlab function ClosedLoop_V1_2020b/MATLAB Function1 ==
  data: switch_signal input; Output output; Input_1 input; Input_2 input
function Output  = fcn(switch_signal, Input_1, Input_2)

if switch_signal == 1
    Output = Input_1;
else
    Output = Input_2;
end

== matlab function ClosedLoop_V1_2020b/MATLAB Function ==
  data: switch_signal input; Output output; Input_1 input; Input_2 input
function Output  = fcn(switch_signal, Input_1, Input_2)

if switch_signal == 1
    Output = Input_1;
else
    Output = Input_2;
end

== matlab function ClosedLoop_V1_2020b/Controller/Rate Saturation Pitch ==
  data: u input; MinSaturation input; y_out output; MaxSaturation input; DT input
function y_out = fcn(u, MinSaturation, MaxSaturation, DT)
persistent y

if isempty(y)
    y = u;
end

rate = (u-y)/DT;
rate = min(max(rate, MinSaturation), MaxSaturation);

y = y + rate*DT;
y_out = y;

== matlab function ClosedLoop_V1_2020b/Controller/Pitch Control/PitchControl ==
  settings: updateMethod=DISCRETE  sampleTime=Control.DT
  data: GeneratorSpeedError input; GeneratorSpeed input; MeasuredTorque input; MeasuredPitch input; BladePitch output; KP input; KI input; MinMaxPitch input; MinMaxPitchRate input; DT input; P_InitAngle input; P_StartupPitch input; GearboxRatio input; P_StartUpSpeed input; P_StartupPitchRate input; omega_C input; Demanded_torque input; Clock input; P_LowRateModeOut output boolean; Event input; EventTime input
function [BladePitch, P_LowRateModeOut]  = PitchControl(GeneratorSpeedError, GeneratorSpeed, MeasuredTorque, MeasuredPitch, KP, KI, MinMaxPitch, MinMaxPitchRate, DT, P_InitAngle, P_StartupPitch, GearboxRatio, P_StartUpSpeed, P_StartupPitchRate, omega_C, Demanded_torque, Clock, Event, EventTime)
persistent I_term PI_term_old P_LowRateMode P_LowRateMode_old

%Initialize all persistent variables
if isempty(I_term)
    I_term = (P_InitAngle*pi/180);
    PI_term_old = (P_InitAngle*pi/180);
    P_LowRateMode = true;
    P_LowRateMode_old = true; %Used to detect change from start-up/below-rated to above-rated operation mode
end

%Event handling part
if (Event == 2 && Clock >= EventTime) || (Event == 5 && Clock >= EventTime) %Grid loss, emergency shutdown
    P_LowRateMode = false;
    P_MinPitchSat = MinMaxPitch(2)*pi/180;
elseif (Event == 4 && Clock >= EventTime) % Normal shutdown
    P_LowRateMode = true;
    P_MinPitchSat = MinMaxPitch(2)*pi/180;
elseif Event == 7 || Event == 6 % Idling and parked mode
    P_MinPitchSat = MinMaxPitch(2)*pi/180;
elseif MeasuredTorque > Demanded_torque*0.99 || GeneratorSpeed > omega_C*(pi/30) % Above-rated operating mode
    P_LowRateMode = false;
    P_MinPitchSat = MinMaxPitch(1)*pi/180;
    if P_LowRateMode ~= P_LowRateMode_old % On switching event between below-rated to above rated, reinitialize the integral term to ensure smooth transition
        I_term = MeasuredPitch;
    end
elseif Event == 3 || GeneratorSpeed < P_StartUpSpeed*GearboxRatio*(pi/30) % Normal startup 
    if Event == 3 && Clock < EventTime
        P_LowRateMode = true;
        P_MinPitchSat = MinMaxPitch(2)*pi/180;
    elseif (Event == 3 && Clock >= EventTime) && (GeneratorSpeed < P_StartUpSpeed*GearboxRatio*(pi/30))
        P_LowRateMode = true;
        P_MinPitchSat = P_StartupPitch*pi/180;
    else
        P_LowRateMode = true;
        P_MinPitchSat = MinMaxPitch(1)*pi/180;
    end
else
    P_MinPitchSat = MinMaxPitch(1)*pi/180;
end
 
% Pitch controller, KP and KI are constant or gain-scheduled, depending on
% input. Integral term is saturated, lower bound is variable and depends on
% event or operatinig mode.
P_term = KP*GeneratorSpeedError;
I_term = I_term + KI*GeneratorSpeedError*DT;
I_term = min(max(I_term,P_MinPitchSat), MinMaxPitch(2)*pi/180);

PI_term = P_term + I_term;
PI_term_sat = min(max(PI_term,P_MinPitchSat), MinMaxPitch(2)*pi/180);

% Calculate and limit pitch rate. Limit on rate is subject to event or
% operating mode.
PitchRate = (PI_term_sat - PI_term_old)/DT;
if P_LowRateMode
    PitchRate = min(max(PitchRate, -P_StartupPitchRate*pi/180), P_StartupPitchRate*pi/180);
else
    PitchRate = min(max(PitchRate, MinMaxPitchRate(1)*pi/180), MinMaxPitchRate(2)*pi/180);
end
BladePitch = PI_term_old + PitchRate*DT;

% Write variables to persistent variables and/or outputs
PI_term_old = BladePitch;
P_LowRateModeOut = P_LowRateMode;
P_LowRateMode_old = P_LowRateMode;
end
